simulink model "mpc_pendcartNMPC"  (R2021a)
settings: Solver=ode15s  StartTime=0.0  StopTime=30  MaxStep=1e-3  RelTol=1e-3  EnableMultiTasking=on
values from neighbouring files (symbols this model uses):
  Ts = 0.2    [SwingupControlOfPendulumNMPC.m]    (also in pendulumStateFcn.m = u(2))
undefined symbols (not defined in the file or in its folder): sigbuilder_block
libraries: mpclib x1, sharedTrackingLibrary x1
settings Model: Creator=The MathWorks, Inc.  LastModifiedBy=The MathWorks, Inc.
settings SolverCC: AlgebraicLoopSolver=LineSearch
settings DataIOCC: LimitDataPoints=on  SaveFormat=Array  ReturnWorkspaceOutputs=off
settings OptimizationCC: LifeSpan=inf
settings DebuggingCC: AlgebraicLoopMsg=none  UnderspecifiedInitializationDetection=Classic  MergeDetectMultiDrivingBlocksExec=none  SolverPrmCheckMsg=warning  AllowSymbolicDim=off  StateNameClashWarn=warning  SFUnexpectedBacktrackingDiag=warning  SFNoUnconditionalDefaultTransitionDiag=warning  SFExecutionAtInitializationDiag=none  SFMachineParentedDataDiag=warning  ArithmeticOperatorsInVariantConditions=warning
settings HardwareCC: ProdBitPerPointer=32  ProdBitPerSizeT=32  ProdBitPerPtrDiffT=32  ProdLargestAtomicFloat=None  ProdIntDivRoundTo=Undefined  ProdEndianess=Unspecified  ProdWordSize=32  ProdHWDeviceType=32-bit Generic
settings ModelReferenceCC: PropagateSignalLabelsOutOfModel=off
settings SFSimCC: SimUseLocalCustomCode=off  CustomCodeUndefinedFunction=UseInterfaceOnly
settings RTWCC: RTWUseLocalCustomCode=off
settings CodeAppCC: StateflowObjectComments=on
settings GRTTargetCC: TargetLangStandard=C89/C90 (ANSI)
settings ConfigComp: CovMetricSettings=dw  CovSaveCumulativeToWorkspaceVar=on  CovSaveSingleToWorkspaceVar=on  CovExternalEMLEnable=off  CovSFcnEnable=off
settings SimscapeCC: SimscapeNormalizeSystem=off  SimscapeNominalValues="[{\"value\":\"10\",\"unit\":\"V\"},{\"value\":\"1\",\"unit\":\"A\"},{\"value\":\"10\",\"unit\":\"N*m\"},{\"value\":\"10\",\"unit\":\"bar\"},{\"value\":\"100\",\"unit\":\"kJ/kg\"},{\"value\":\"1\",\"unit\":\"kW\"},{\"value\":\"300\",\"unit\":\"K\"},{\"value\":\"100\",\"unit\":\"cm^3/s\"},{\"value\":\"1\",\"unit\":\"kN\"},{\"value\":\"1\",\"unit\":\"g/cm^3\"},{\"value\":\"1\",\"unit\":\"l\"},{\"value\":\"1\",\"unit\":\"cm^2\"},{\"value\":\"60\",\"unit\":\"Hz\"}]"
settings ConfigurationSet: Description=SimMechanics 2G
settings ExplorerConfigSet: InternalSimMechanicsExplorerSettings="<ExplorerConfiguration><canonicalview>default</canonicalview><AnimationSetting><BasePlaybackSpeed>1.0</BasePlaybackSpeed><PlaybackSpeedFactor>1.0</PlaybackSpeedFactor></AnimationSetting><TilePanel><TileInfo><Tiles Columns=\"1\" Count=\"1\" Rows=\"1\"><Column Left=\"2\" Weight=\"1\"/><Column Left=\"1552\"/><Row Top=\"2\" Weight=\"1\"/><Row Top=\"932\"/><Tile Height=\"1\" Width=\"1\" X=\"0\" Y=\"0\"/></Tiles></TileInfo><SceneInfo><SceneViewer><BGColor><R>0.60000002384185791</R><G>0.60000002384185791</G><B>0.60000002384185791</B></BGColor><Camera><Position><X>0.027865189060748197</X><Y>-2.5719092456962986</Y><Z>0.23157896538506753</Z></Position><Center><X>0.62659712312732463</X><Y>-0.46110119691712204</Y><Z>0.22087365386473376</Z></Center><Up><X>-0.0079438354874226333</X><Y>0.0073246425924307582</Y><Z>0.99994162084025784</Z></Up><Left>-0.24533778208815546</Left><Right>0.24533778208815546</Right><Bottom>-0.79734779727023208</Bottom><Top>0.79734779727023208</Top></Camera></SceneViewer></SceneInfo></TilePanel></ExplorerConfiguration>"

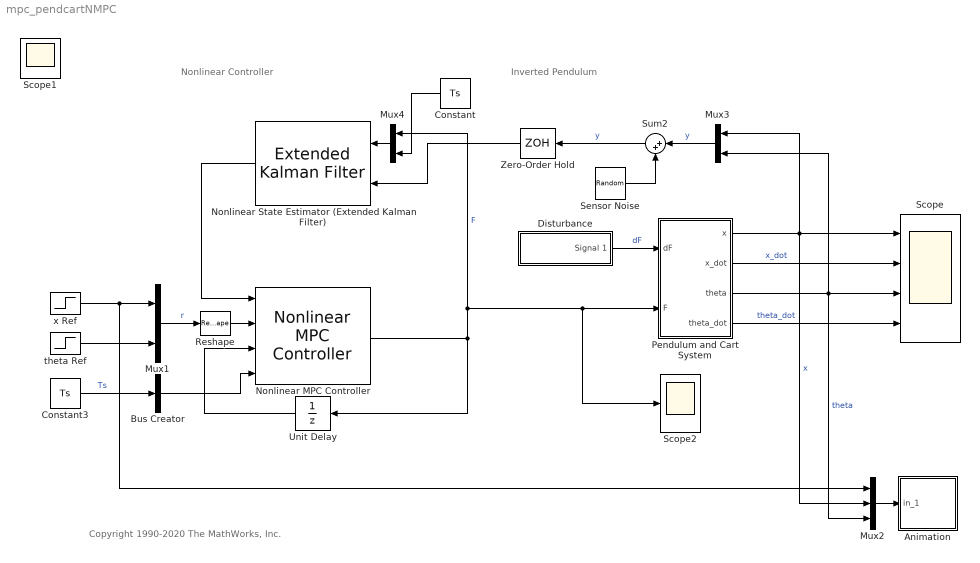
== system mpc_pendcartNMPC ==
  note: Nonlinear Controller
  note: Copyright 1990-2020 The MathWorks, Inc.
  note: Inverted Pendulum
  Animation : Subsystem  mask(Pendulum plot){RefBlock=x Ref}
      mask prompts: RefBlock "Cart Reference Signal Block Name:"
      mask help: Pendulum plot
      mask Help: Pendulum animation function using Handle graphics.
      mask Display: plot([-10 10],[0 0],[-2 -2 2 2],[0 1 1 0],[0 3],[1 5])
  Bus Creator : BusCreator  Inputs=1  OutDataTypeStr=Bus: myBusObject  NonVirtualBus=on
      settings: InheritFromInputs=off
  Constant : Constant  Value=Ts
  Constant3 : Constant  Value=Ts
  Disturbance : Subsystem  Tag=STV Subsys  LoadFcn=sigbuilder_block('load');  StartFcn=sigbuilder_block('start');  StopFcn=sigbuilder_block('stop');  ClipboardFcn=sigbuilder_block('clipboard');  mask(Sigbuilder block){tuvar=[0:10]}
      mask help: Simulink:masks:SigbuilderBlock_MD
      mask init:
      | if ~strcmp(get_param(bdroot(gcbh),'SimulationStatus'),'stopped') tuvar = sigbuilder_block('maskInit'); end
      settings: CopyFcn=sigbuilder_block('copy');  DeleteFcn=sigbuilder_block('delete');  ModelCloseFcn=sigbuilder_block('modelClose');  PreSaveFcn=sigbuilder_block('preSave');  PauseFcn=sigbuilder_block('pause');  ContinueFcn=sigbuilder_block('continue');  NameChangeFcn=sigbuilder_block('namechange');  OpenFcn=sigbuilder_block('open',[237 187.5 551.25 396 ]);  CloseFcn=sigbuilder_block('close');
      mask Display: plot(0, 0, 100, 100,[2, 2, 32, 32, 2], [68, 8, 8, 68, 68],[32, 2], [38, 38], [32, 19, 2],[53, 60, 44], [32, 17, 17, 2],[16, 16, 31, 31]);txt = getActiveGroup(gcbh);text(2, 100, txt,'verticalAlignment', 'top');
  Mux1 : Mux  Inputs=2
  Mux2 : Mux  Inputs=3
  Mux3 : Mux  Inputs=2
  Mux4 : Mux  Inputs=2
  Nonlinear MPC Controller : mpclib/Nonlinear MPC Controller  SCDEnableBlockLinearizationSpecification=on  nlmpcobj=nlobj  UseObjectTs=on  UseMEX=off  md_enabled=off  mvtarget_enabled=off  param_enabled=on  cost_enabled=off  mvseq_enabled=off  stateseq_enabled=off  ovseq_enabled=off  slack_enabled=off  status_enabled=off  ov_min=off  ov_max=off  mv_min=off  mv_max=off  mvrate_min=off  mvrate_max=off  state_min=off  state_max=off  ov_weight=off  mv_weight=off  mvrate_weight=off  ecr_weight=off  nlp_initialize=off
  Nonlinear State Estimator (Extended Kalman Filter) : sharedTrackingLibrary/Extended Kalman Filter  StateTransitionFcn=pendulumStateFcn  HasStateTransitionJacobianFcn=off  HasAdditiveProcessNoise=Additive  ProcessNoise=1e-4*eye(4)  HasTimeVaryingProcessNoise=off  HasStateTransitionFcnExtraArgument=1  InitialState=[0;0;-pi;0]  InitialStateCovariance=1e-4*eye(4)  MeasurementFcn1=pendulumMeasurementFcn  HasMeasurementJacobianFcn1=off  HasMeasurementEnablePort1=off  HasAdditiveMeasurementNoise1=Additive  MeasurementNoise1=1e-4*eye(2)  HasTimeVaryingMeasurementNoise1=off  HasMeasurementFcnExtraArgument1=0  MeasurementFcn2=myMeasurementFcn  HasMeasurementJacobianFcn2=off  HasMeasurementEnablePort2=off  HasAdditiveMeasurementNoise2=Additive  MeasurementNoise2=1  HasTimeVaryingMeasurementNoise2=off  HasMeasurementFcnExtraArgument2=0  MeasurementFcn3=myMeasurementFcn  HasMeasurementJacobianFcn3=off  HasMeasurementEnablePort3=off  HasAdditiveMeasurementNoise3=Additive  MeasurementNoise3=1  HasTimeVaryingMeasurementNoise3=off  HasMeasurementFcnExtraArgument3=0  MeasurementFcn4=myMeasurementFcn  HasMeasurementJacobianFcn4=off  HasMeasurementEnablePort4=off  HasAdditiveMeasurementNoise4=Additive  MeasurementNoise4=1  HasTimeVaryingMeasurementNoise4=off  HasMeasurementFcnExtraArgument4=0  MeasurementFcn5=myMeasurementFcn  HasMeasurementJacobianFcn5=off  HasMeasurementEnablePort5=off  HasAdditiveMeasurementNoise5=Additive  MeasurementNoise5=1  HasTimeVaryingMeasurementNoise5=off  HasMeasurementFcnExtraArgument5=0  EnableMultirate=off  StateTransitionFcnSampleTime=1  MeasurementFcn1SampleTime=1  MeasurementFcn2SampleTime=1  MeasurementFcn3SampleTime=1  MeasurementFcn4SampleTime=1  MeasurementFcn5SampleTime=1  UseCurrentEstimator=on  OutputStateCovariance=off  DataType=double  SampleTime=Ts  NumberOfMeasurements=1
      settings: SourceProductBaseCode=CT,DR,TF,ID,LP,NV,AR,RO,RR,UV,VE
  Pendulum and Cart System : Subsystem  mask{mCartPara=1, mPendPara=1, gPara=9.81, LPara=0.5, KdPara=10, x0=0, theta0=-pi}
      mask prompts: mCartPara "Mass of Cart"; mPendPara "Mass of Pendulum"; gPara "Gravity"; LPara "Length of Pendulum"; KdPara "Friction coefficient of Cart"; x0 "Initial Cart Position"; theta0 "Initial Pendulum Angle"
      mask help: Pendulum and Cart System
      mask init:
      | mCart = str2double(get_param(gcb,'mCartPara'));
      | mPend = str2double(get_param(gcb,'mPendPara'));
      | g = str2double(get_param(gcb,'gPara'));
      | L = str2double(get_param(gcb,'LPara'));
      | Kd = str2double(get_param(gcb,'KdPara'));
  Reshape : Reshape  OutputDimensionality=Row vector (2-D)
  Scope : Scope  NumInputPorts=4
  Scope2 : Scope
  Sensor Noise : UniformRandomNumber  Minimum=-0.01  Maximum=0.01  SampleTime=Ts
  Sum2 : Sum  Inputs=|++
  Unit Delay : UnitDelay  SampleTime=-1  HasFrameUpgradeWarning=on
  Zero-Order Hold : ZeroOrderHold  SampleTime=Ts
  theta Ref : Step  Before=-pi  After=0  SampleTime=0
  x Ref : Step  Time=10  After=5  SampleTime=0
  Scope1 : Scope
  wires:
  theta Ref/1 -> Mux1/2
  Pendulum and Cart System/4(theta_dot) -> Scope/4  "theta_dot"
  Pendulum and Cart System/2(x_dot) -> Scope/2  "x_dot"
  Disturbance/1(Signal 1) -> Pendulum and Cart System/1(dF)  "dF"
  Nonlinear MPC Controller/1 -> Unit Delay/1, Pendulum and Cart System/2(F), Scope2/1, Mux4/1  "F"
  Mux2/1 -> Animation/1(in_1)
  x Ref/1 -> Mux2/1, Mux1/1
  Unit Delay/1 -> Nonlinear MPC Controller/3
  Mux3/1 -> Sum2/1  "y"
  Sensor Noise/1 -> Sum2/2
  Pendulum and Cart System/3(theta) -> Mux3/2, Mux2/3, Scope/3  "theta"
  Sum2/1 -> Zero-Order Hold/1  "y"
  Pendulum and Cart System/1(x) -> Mux3/1, Mux2/2, Scope/1  "x"
  Zero-Order Hold/1 -> Nonlinear State Estimator (Extended Kalman Filter)/2
  Mux4/1 -> Nonlinear State Estimator (Extended Kalman Filter)/1
  Constant/1 -> Mux4/2
  Nonlinear State Estimator (Extended Kalman Filter)/1 -> Nonlinear MPC Controller/1
  Mux1/1 -> Reshape/1  "r"
  Reshape/1 -> Nonlinear MPC Controller/2
  Constant3/1 -> Bus Creator/1  "Ts"
  Bus Creator/1 -> Nonlinear MPC Controller/4

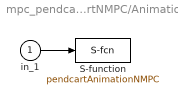
== system mpc_pendcartNMPC/Animation ==
  in_1 : Inport
  S-function : S-Function  FunctionName=pendcartAnimationNMPC  Parameters=RefBlock  SFunctionDeploymentMode=off  EnableBusSupport=off
      settings: DeleteFcn=pendcartAnimationNMPC([],[],[],'DeleteBlock');
  wires:
  in_1/1 -> S-function/1

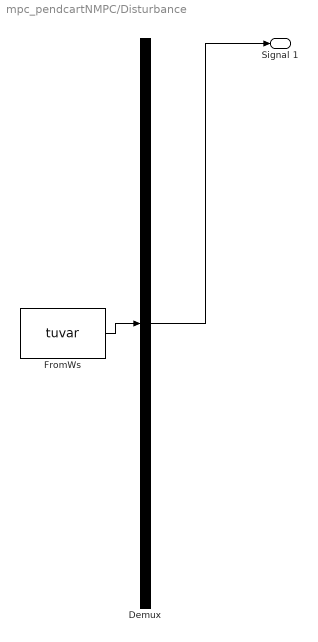
== system mpc_pendcartNMPC/Disturbance ==
  Demux : Demux  Tag=STV Demux  Outputs=1
      settings: DisplayOption=none
  FromWs : FromWorkspace  Tag=STV FromWs  VariableName=tuvar
      SigBuilderData=|
      | common.afterFinalStr = 'Extrapolate'
      | common.sampleTime = 0
      | dataSet.timeRange = [0 30]
      | dataSet.name = 'Group 1'
      | sbobj.Groups.Name = 'Group 1'
      | sbobj.Groups.Signals.Name = 'Signal 1'
      | sbobj.Groups.Signals.XData = [0 20 20.5 21 30]
      | sbobj.Groups.Signals.YData = [0 0 2 0 0]
      | sbobj.Groups.TimeRange = [0 30]
  Signal 1 : Outport  Tag=STV Outport  VectorParamsAs1DForOutWhenUnconnected=off
  wires:
  FromWs/1 -> Demux/1
  Demux/1 -> Signal 1/1

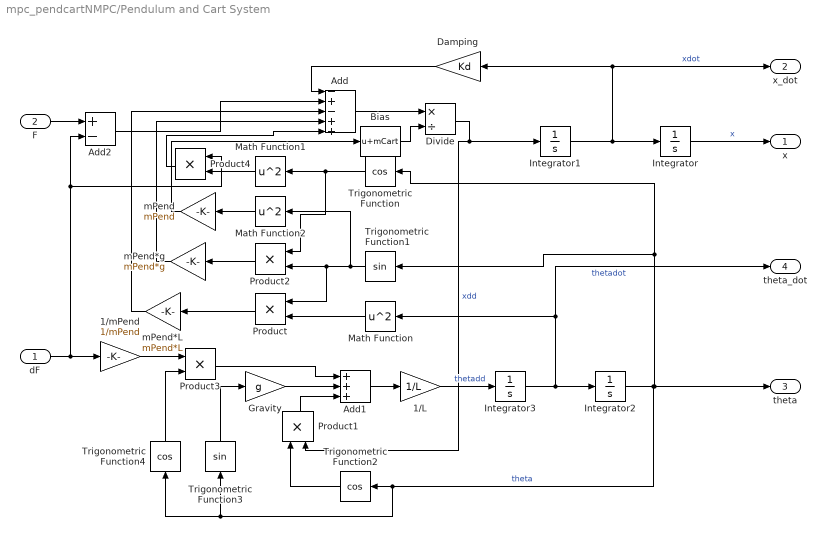
== system mpc_pendcartNMPC/Pendulum and Cart System ==
  dF : Inport
  F : Inport  Port=2
  1/L : Gain  Gain=1/L
  1/mPend : Gain  Gain=1/mPend
  Add : Sum  Inputs=-+-++
  Add1 : Sum  Inputs=+++
  Add2 : Sum  Inputs=+-
  Bias : Bias  Bias=mCart
  Damping : Gain  Gain=Kd
  Divide : Product  Inputs=*/
  Gravity : Gain  Gain=g
  Integrator : Integrator  InitialCondition=x0  ContinuousStateAttributes='x'
  Integrator1 : Integrator  ContinuousStateAttributes='xdot'
  Integrator2 : Integrator  InitialCondition=theta0  ContinuousStateAttributes='theta'
  Integrator3 : Integrator  ContinuousStateAttributes='thetadot'
  Math Function : Math  Operator=square  SignedPower=on  SaturateOnIntegerOverflow=on
  Math Function1 : Math  Operator=square  SignedPower=on  SaturateOnIntegerOverflow=on
  Math Function2 : Math  Operator=square  SignedPower=on  SaturateOnIntegerOverflow=on
  Product{,1..4} (5 alike) : Product
  Trigonometric Function : Trigonometry  Operator=cos
  Trigonometric Function1 : Trigonometry
  Trigonometric Function2 : Trigonometry  Operator=cos
  Trigonometric Function3 : Trigonometry
  Trigonometric Function4 : Trigonometry  Operator=cos
  mPend : Gain  Gain=mPend
  mPend*L : Gain  Gain=mPend*L
  mPend*g : Gain  Gain=mPend*g
  x : Outport  VectorParamsAs1DForOutWhenUnconnected=off
  x_dot : Outport  Port=2  VectorParamsAs1DForOutWhenUnconnected=off
  theta : Outport  Port=3  VectorParamsAs1DForOutWhenUnconnected=off
  theta_dot : Outport  Port=4  VectorParamsAs1DForOutWhenUnconnected=off
  wires:
  mPend/1 -> Bias/1
  Bias/1 -> Divide/2
  Math Function2/1 -> mPend/1
  Product4/1 -> Add/5
  Math Function1/1 -> Product4/2
  mPend*g/1 -> Add/4
  Product1/1 -> Add1/3
  Math Function/1 -> Product/2
  1/L/1 -> Integrator3/1  "thetadd"
  dF/1 -> 1/mPend/1, Product4/1, Add2/2
  1/mPend/1 -> Product3/1
  Trigonometric Function4/1 -> Product3/2
  Damping/1 -> Add/1
  F/1 -> Add2/1
  Trigonometric Function3/1 -> Gravity/1
  Gravity/1 -> Add1/2
  Trigonometric Function/1 -> Math Function1/1, Product2/1
  Integrator3/1 -> Integrator2/1, Math Function/1, theta_dot/1  "thetadot"
  Integrator2/1 -> Trigonometric Function2/1, Trigonometric Function3/1, Trigonometric Function4/1, Trigonometric Function1/1, Trigonometric Function/1, theta/1  "theta"
  Product3/1 -> Add1/1
  Add/1 -> Divide/1
  Divide/1 -> Integrator1/1, Product1/2  "xdd"
  Trigonometric Function2/1 -> Product1/1
  Trigonometric Function1/1 -> Math Function2/1, Product/1, Product2/2
  Integrator/1 -> x/1  "x"
  Integrator1/1 -> Damping/1, x_dot/1, Integrator/1  "xdot"
  Product2/1 -> mPend*g/1
  Add1/1 -> 1/L/1
  Add2/1 -> Add/2
  mPend*L/1 -> Add/3
  Product/1 -> mPend*L/1
